simulink model "Velo"  (R2018a)
settings: Solver=ode15s  StartTime=0.0  StopTime=10.0  FixedStep=0.0001  RelTol=1e-3
model mask{InitialCondition=5}
  mask prompts: InitialCondition "Angle initial"
model workspace (MAT data in the model file):
  InitialCondition = 5
undefined symbols (not defined in the file): g, Jr, Jv, Lr, Lv, Mr, Mv
settings Model: ParameterArgumentNames=InitialCondition  Creator=chsira  LastModifiedBy=charl
settings DataIOCC: SaveOutput=off  SignalLogging=off  SaveTime=off
settings DebuggingCC: LibraryContextMissingDiagnostic=warning
settings SFSimCC: SimUseLocalCustomCode=on
settings RTWCC: RTWUseLocalCustomCode=on

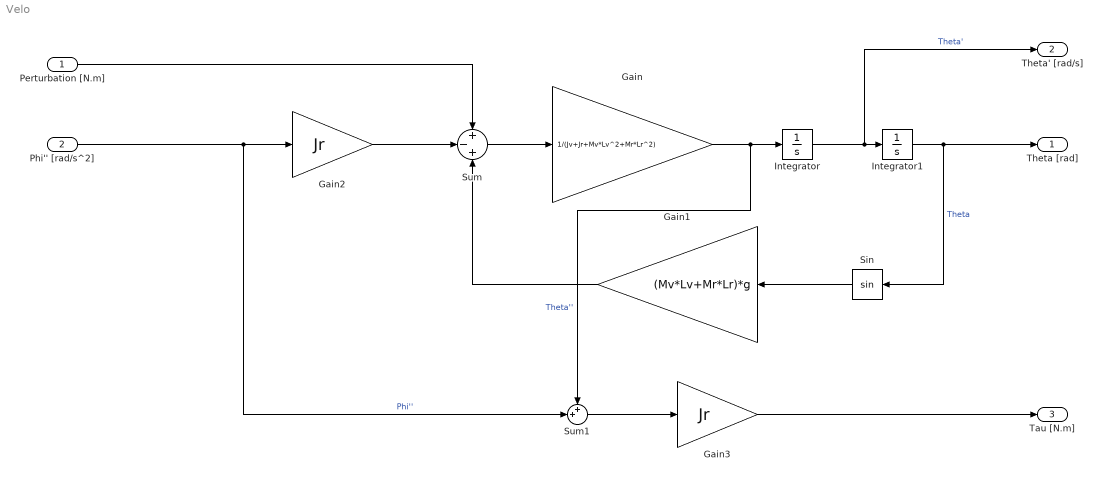
== system Velo ==
  Perturbation [N.m] : Inport  OutDataTypeStr=double  PortDimensions=1  SampleTime=0
  Phi'' [rad/s^2] : Inport  Port=2  OutDataTypeStr=double  PortDimensions=1  SampleTime=0
  Gain : Gain  Gain=1/(Jv+Jr+Mv*Lv^2+Mr*Lr^2)
  Gain1 : Gain  Gain=(Mv*Lv+Mr*Lr)*g
  Gain2 : Gain  Gain=Jr
  Gain3 : Gain  Gain=Jr
  Integrator : Integrator
  Integrator1 : Integrator  InitialCondition=InitialCondition  mask{InitialCondition=InitialCondition}
      mask prompts: InitialCondition "Angle initial"
      mask TypeOptions InitialCondition: InitialCondition
  Sin : Trigonometry
  Sum : Sum  Inputs=+-+
  Sum1 : Sum  Inputs=++|
  Theta [rad] : Outport  OutDataTypeStr=double  PortDimensions=1  SampleTime=0
  Theta' [rad/s] : Outport  Port=2  OutDataTypeStr=double  PortDimensions=1  SampleTime=0
  "Tau [N.m] " : Outport  Port=3  OutDataTypeStr=double  PortDimensions=1  SampleTime=0
  wires:
  Sin/1 -> Gain1/1
  Gain/1 -> Integrator/1, Sum1/1  "Theta''"
  Gain1/1 -> Sum/3
  Integrator/1 -> Theta' [rad/s]/1, Integrator1/1  "Theta'"
  Gain2/1 -> Sum/2
  Sum/1 -> Gain/1
  Integrator1/1 -> Theta [rad]/1, Sin/1  "Theta"
  Phi'' [rad/s^2]/1 -> Gain2/1, Sum1/2  "Phi''"
  Sum1/1 -> Gain3/1
  Gain3/1 -> "Tau [N.m] "/1
  Perturbation [N.m]/1 -> Sum/1
